simulink model "TorqueVect"  (R2022a)
settings: Solver=VariableStepAuto  StartTime=0.0  StopTime=300  RelTol=1e-3
PreLoadFcn:
  | run('Parameters\FSE_Parameters.m')
values from neighbouring files (symbols this model uses):
  Kd = 0;')    [open_carmaker_gui.m]
  Ki = 0    [open_carmaker_gui.m]
undefined symbols (not defined in the file or in its folder): BRegenEnabledButton, canChannel, CyalphaLookUp, efficiency, Fz_curve, Fz_scaling_long, gearR, izz, jw, kd, ki, Kp, kp, l_f, l_r, lambda, m, Mz_max, N, N_lat, N_long, P_max, pid_kd_lat, pid_kd_long, pid_ki_lat, pid_ki_long, pid_kp_lat, pid_kp_long, R_max, rw, steerR, T_i_max, TC_Decr_Gas, TC_Derivative, TC_Incr_Gas, TC_On, TC_Relay_Off, TC_Relay_On, tireCornerStiffness, Ts, TV_On, TV_Override, velocity_lookup, velocity_lookup_lat, y_ref, yrr_scaling
libraries: simulink x218, slpidlib x135, CarMaker4SL x73, TractionControlLibrary x13, canmsglib x9, canlib x8, TorqueVectoringLibrary x6, simulink_extras x4, PedalConversionLibrary x3, PowerControlLibrary x1
(part 7 of 26)

== system TorqueVect/CarMaker/IPG Vehicle/PowerTrain/PTControl Example/PTControl_ALL_CTRL_VC_MFE24/New TC/TC R3 ==
  modified slip ratio reference : Inport
  lim 1 : Inport  Port=2
  modified slip ratio measurement : Inport  Port=3
  P_TC : Inport  Port=4
  D_TC : Inport  Port=5
  enable_tc : Inport  Port=6
  PID Controller : slpidlib/PID Controller  Commented=on  Controller=PD  Form=Parallel  TimeDomain=Discrete-time  UseExternalTs=off  SampleTime=-1  IntegratorMethod=Forward Euler  FilterMethod=Forward Euler  ControllerParametersSource=external  P=125  I=1  UseKiTs=on  D=0  N=100  UseFilter=on  TunerSelectOption=Transfer Function Based (PID Tuner App)  InitialConditionSource=internal  InitialConditionForIntegrator=0  InitialConditionForFilter=0  DifferentiatorICPrevScaledInput=0  ExternalReset=none  TrackingMode=off  Kt=1  LimitOutput=on  SatLimitsSource=external  UpperSaturationLimit=inf  LowerSaturationLimit=-inf  LinearizeAsGain=on  AntiWindupMode=clamping  Kb=1  POutMin=[]  POutMax=[]  IOutMin=[]  IOutMax=[]  DOutMin=[]  DOutMax=[]  NOutMin=[]  NOutMax=[]  SumOutMin=[]  SumOutMax=[]  SaturationOutMin=[]  SaturationOutMax=[]  PParamMin=[]  PParamMax=[]  IParamMin=[]  IParamMax=[]  DParamMin=[]  DParamMax=[]  NParamMin=[]  NParamMax=[]  KbParamMin=[]  KbParamMax=[]  KtParamMin=[]  KtParamMax=[]  KbOutMin=[]  KbOutMax=[]  KtOutMin=[]  KtOutMax=[]  IntegratorOutMin=[]  IntegratorOutMax=[]  FilterOutMin=[]  FilterOutMax=[]  SumI1OutMin=[]  SumI1OutMax=[]  SumI2OutMin=[]  SumI2OutMax=[]  SumI3OutMin=[]  SumI3OutMax=[]  SumI4OutMin=[]  SumI4OutMax=[]  SumDOutMin=[]  SumDOutMax=[]  DifferentiatorOutMin=[]  DifferentiatorOutMax=[]  FilterDiffOutCoefMin=[]  FilterDiffOutCoefMax=[]  ReciprocalOutMin=[]  ReciprocalOutMax=[]  SumDenOutMin=[]  SumDenOutMax=[]  SumNumOutMin=[]  SumNumOutMax=[]  DivideOutMin=[]  DivideOutMax=[]  UdiffTsProdOutMin=[]  UdiffTsProdOutMax=[]  NTsProdOutMin=[]  NTsProdOutMax=[]  UintegralTsProdOutMin=[]  UintegralTsProdOutMax=[]  UngainTsProdOutMin=[]  UngainTsProdOutMax=[]  ClampingZeroOutDataTypeStr=Inherit: Inherit via back propagation  ClampingZeroOutMin=[]  ClampingZeroOutMax=[]  FilterDenConstantOutDataTypeStr=Inherit: Inherit via back propagation  FilterDenConstantOutMin=[]  FilterDenConstantOutMax=[]  PCopyOutDataTypeStr=Inherit: Inherit via back propagation  PCopyOutMin=[]  PCopyOutMax=[]  NCopyOutDataTypeStr=Inherit: Inherit via back propagation  NCopyOutMin=[]  NCopyOutMax=[]  IntegratorContinuousStateAttributes=''  IntegratorStateMustResolveToSignalObject=off  IntegratorRTWStateStorageClass=Auto  FilterContinuousStateAttributes=''  FilterStateMustResolveToSignalObject=off  FilterRTWStateStorageClass=Auto  ParallelPVariant=ExternalParameters  IdealPVariant=Disabled  IVariant=Disabled  DVariant=ExternalParameters  IntegratorVariant=Disabled  SatVariant=External  AWVariant=Disabled  PCopyVariant=Disabled  TRVariant=Disabled  FdbkBlocksVariant=Forward  IdealPFdbkVariant=Disabled  SatFdbkVariant=Disabled  DerivativeFilterVariant=ForwardEulerFilter  NVariant=ExternalParameters  NCopyVariant=Disabled  FilterICVariant=InternalICsFilter  IntegratorICVariant=Disabled  ExternalResetVariant=Disabled  TRSumVariant=Passthrough  SumFdbkVariant=Disabled  SumVariant=Sum_PD  TsampFilterVariant=InternalTs  TsampNgainVariant=Passthrough  TsampIntegralVariant=Disabled_SignalSpec  ExternalSaturationOutDataTypeStr=Inherit: Same as second input  aMode=0
  Sum1 : Sum  Inputs=|-+
  Sum2 : Sum  Commented=on  Inputs=|-+
  traction_controller : Subsystem
  Control Effort 1 : Outport
  wires:
  modified slip ratio reference/1 -> Sum1/1
  modified slip ratio measurement/1 -> Sum1/2
  lim 1/1 -> Sum2/2, traction_controller/1(max_torque)
  PID Controller/1 -> Sum2/1
  traction_controller/1(delta_torque) -> Control Effort 1/1
  enable_tc/1 -> traction_controller/3(enable_tc)
  Sum1/1 -> traction_controller/2(dslip)
  P_TC/1 -> traction_controller/4(Kp)
  D_TC/1 -> traction_controller/5(Kd)

== system TorqueVect/CarMaker/IPG Vehicle/PowerTrain/PTControl Example/PTControl_ALL_CTRL_VC_MFE24/New TC/TC R4 ==
  modified slip ratio reference : Inport
  lim 1 : Inport  Port=2
  modified slip ratio measurement : Inport  Port=3
  P_TC : Inport  Port=4
  D_TC : Inport  Port=5
  enable_tc : Inport  Port=6
  PID Controller : slpidlib/PID Controller  Commented=on  Controller=PD  Form=Parallel  TimeDomain=Discrete-time  UseExternalTs=off  SampleTime=-1  IntegratorMethod=Forward Euler  FilterMethod=Forward Euler  ControllerParametersSource=external  P=125  I=1  UseKiTs=on  D=0  N=100  UseFilter=on  TunerSelectOption=Transfer Function Based (PID Tuner App)  InitialConditionSource=internal  InitialConditionForIntegrator=0  InitialConditionForFilter=0  DifferentiatorICPrevScaledInput=0  ExternalReset=none  TrackingMode=off  Kt=1  LimitOutput=on  SatLimitsSource=external  UpperSaturationLimit=inf  LowerSaturationLimit=-inf  LinearizeAsGain=on  AntiWindupMode=clamping  Kb=1  POutMin=[]  POutMax=[]  IOutMin=[]  IOutMax=[]  DOutMin=[]  DOutMax=[]  NOutMin=[]  NOutMax=[]  SumOutMin=[]  SumOutMax=[]  SaturationOutMin=[]  SaturationOutMax=[]  PParamMin=[]  PParamMax=[]  IParamMin=[]  IParamMax=[]  DParamMin=[]  DParamMax=[]  NParamMin=[]  NParamMax=[]  KbParamMin=[]  KbParamMax=[]  KtParamMin=[]  KtParamMax=[]  KbOutMin=[]  KbOutMax=[]  KtOutMin=[]  KtOutMax=[]  IntegratorOutMin=[]  IntegratorOutMax=[]  FilterOutMin=[]  FilterOutMax=[]  SumI1OutMin=[]  SumI1OutMax=[]  SumI2OutMin=[]  SumI2OutMax=[]  SumI3OutMin=[]  SumI3OutMax=[]  SumI4OutMin=[]  SumI4OutMax=[]  SumDOutMin=[]  SumDOutMax=[]  DifferentiatorOutMin=[]  DifferentiatorOutMax=[]  FilterDiffOutCoefMin=[]  FilterDiffOutCoefMax=[]  ReciprocalOutMin=[]  ReciprocalOutMax=[]  SumDenOutMin=[]  SumDenOutMax=[]  SumNumOutMin=[]  SumNumOutMax=[]  DivideOutMin=[]  DivideOutMax=[]  UdiffTsProdOutMin=[]  UdiffTsProdOutMax=[]  NTsProdOutMin=[]  NTsProdOutMax=[]  UintegralTsProdOutMin=[]  UintegralTsProdOutMax=[]  UngainTsProdOutMin=[]  UngainTsProdOutMax=[]  ClampingZeroOutDataTypeStr=Inherit: Inherit via back propagation  ClampingZeroOutMin=[]  ClampingZeroOutMax=[]  FilterDenConstantOutDataTypeStr=Inherit: Inherit via back propagation  FilterDenConstantOutMin=[]  FilterDenConstantOutMax=[]  PCopyOutDataTypeStr=Inherit: Inherit via back propagation  PCopyOutMin=[]  PCopyOutMax=[]  NCopyOutDataTypeStr=Inherit: Inherit via back propagation  NCopyOutMin=[]  NCopyOutMax=[]  IntegratorContinuousStateAttributes=''  IntegratorStateMustResolveToSignalObject=off  IntegratorRTWStateStorageClass=Auto  FilterContinuousStateAttributes=''  FilterStateMustResolveToSignalObject=off  FilterRTWStateStorageClass=Auto  ParallelPVariant=ExternalParameters  IdealPVariant=Disabled  IVariant=Disabled  DVariant=ExternalParameters  IntegratorVariant=Disabled  SatVariant=External  AWVariant=Disabled  PCopyVariant=Disabled  TRVariant=Disabled  FdbkBlocksVariant=Forward  IdealPFdbkVariant=Disabled  SatFdbkVariant=Disabled  DerivativeFilterVariant=ForwardEulerFilter  NVariant=ExternalParameters  NCopyVariant=Disabled  FilterICVariant=InternalICsFilter  IntegratorICVariant=Disabled  ExternalResetVariant=Disabled  TRSumVariant=Passthrough  SumFdbkVariant=Disabled  SumVariant=Sum_PD  TsampFilterVariant=InternalTs  TsampNgainVariant=Passthrough  TsampIntegralVariant=Disabled_SignalSpec  ExternalSaturationOutDataTypeStr=Inherit: Same as second input  aMode=0
  Sum1 : Sum  Inputs=|-+
  Sum2 : Sum  Commented=on  Inputs=|-+
  traction_controller : Subsystem
  Control Effort 1 : Outport
  wires:
  modified slip ratio reference/1 -> Sum1/1
  modified slip ratio measurement/1 -> Sum1/2
  lim 1/1 -> Sum2/2, traction_controller/1(max_torque)
  PID Controller/1 -> Sum2/1
  traction_controller/1(delta_torque) -> Control Effort 1/1
  enable_tc/1 -> traction_controller/3(enable_tc)
  Sum1/1 -> traction_controller/2(dslip)
  P_TC/1 -> traction_controller/4(Kp)
  D_TC/1 -> traction_controller/5(Kd)

== system TorqueVect/CarMaker/IPG Vehicle/PowerTrain/PTControl Example/PTControl_ALL_CTRL_VC_MFE24/Subsystem/PedalConversion ==
  rThrottlePedal : Inport  OutMin=0  OutMax=1  PortDimensions=1
      settings: AttributesFormatString=[%<OutMin>, %<OutMax>]
  rLimitThrottleHigh : Inport  Port=2
  rLimitThrottleLow : Inport  Port=3
  BRegenEnable : Inport  Port=4
  vLong : Inport  Port=5
  1-D Lookup Table : Lookup_n-D  NumberOfTableDimensions=1  BreakpointsForDimension1=[0 0.3 0.35 1]  Table=[-1 0 0 1]  InternalRulePriority=Speed  RndMeth=Simplest
  AND : Logic  IconShape=distinctive  AllPortsSameDT=off  OutDataTypeStr=boolean
  Compare To Constant : simulink/Logic and Bit Operations/Compare To Constant  relop=>  const=5.0  OutDataTypeStr=boolean
  Rate Limiter Dynamic : simulink/Discontinuities/Rate Limiter Dynamic
  Saturation : Saturate  UpperLimit=1  LowerLimit=-1  OutMin=-1  OutMax=1
      settings: AttributesFormatString=[%<LowerLimit>, %<UpperLimit>]
  Saturation1 : Saturate  UpperLimit=1  LowerLimit=0  OutMin=-1  OutMax=1
      settings: AttributesFormatString=[%<LowerLimit>, %<UpperLimit>]
  Switch : Switch  Criteria=u2 > Threshold  SaturateOnIntegerOverflow=off  InputSameDT=off
  rThrottle : Outport  OutMin=-1  OutMax=1
      settings: AttributesFormatString=[%<OutMin>, %<OutMax>]
  wires:
  rLimitThrottleHigh/1 -> Rate Limiter Dynamic/1
  rLimitThrottleLow/1 -> Rate Limiter Dynamic/3
  Saturation/1 -> Switch/1
  Saturation1/1 -> Switch/3
  Switch/1 -> rThrottle/1
  rThrottlePedal/1 -> Rate Limiter Dynamic/2
  1-D Lookup Table/1 -> Saturation/1, Saturation1/1
  Rate Limiter Dynamic/1 -> 1-D Lookup Table/1
  AND/1 -> Switch/2
  BRegenEnable/1 -> AND/1
  vLong/1 -> Compare To Constant/1
  Compare To Constant/1 -> AND/2

== system TorqueVect/CarMaker/IPG Vehicle/PowerTrain/PTControl Example/PTControl_ALL_CTRL_VC_MFE24/Subsystem/PowerControl1 ==
  PMeasured : Inport  OutMin=-250000  OutMax=250000  Unit=W  PortDimensions=1
      settings: AttributesFormatString=[%<OutMin>, %<OutMax>] %<Unit>
  rSplitF : Inport  Port=2  OutMin=0  OutMax=1  PortDimensions=1
      settings: AttributesFormatString=[%<OutMin>, %<OutMax>]
  rThrottlePedal : Inport  Port=3  OutMin=0  OutMax=1  PortDimensions=1
      settings: AttributesFormatString=[%<OutMin>, %<OutMax>]
  PLimit : Inport  Port=4  OutMin=0  OutMax=80000  Unit=W  PortDimensions=1
      settings: AttributesFormatString=[%<OutMin>, %<OutMax>] %<Unit>
  FF_PC : Inport  Port=5
  P_PC : Inport  Port=6
  D_PC : Inport  Port=7
  I_PC : Inport  Port=8
  MMotorMax : Inport  Port=9
  rThrottle : Inport  Port=10
  FF_RC : Inport  Port=11
  PRegenLimit : Inport  Port=12
  BRegenEnable : Inport  Port=13
  P_RC : Inport  Port=14
  D_RC : Inport  Port=15
  I_RC : Inport  Port=16
  MRegenMotorMax : Inport  Port=17
  Add : Sum
  Constant : Constant  Value=0
  Constant1 : Constant  Value=0
  Gain : Gain  Gain=0.5
  Gain1 : Gain  Gain=0.5
  PC PID : Subsystem
  PID1 : Subsystem  Commented=on
  PowerError : Subsystem
  RC PID : Subsystem
  RegenError : Subsystem
  ResetPID_PC : Subsystem
  ResetPID_RC : Subsystem
  Subsystem : Subsystem
  TotalPower : Subsystem
  Unit Delay : UnitDelay  SampleTime=-1  HasFrameUpgradeWarning=on
  Unit Delay1 : UnitDelay  SampleTime=-1  HasFrameUpgradeWarning=on
  MChangeMotorFL : Outport  OutMin=-21  OutMax=21  Unit=N*m  PortDimensions=1
      settings: AttributesFormatString=[%<OutMin>, %<OutMax>] %<Unit>
  MChangeMotorFR : Outport  Port=2  OutMin=-21  OutMax=21  Unit=N*m  PortDimensions=1
      settings: AttributesFormatString=[%<OutMin>, %<OutMax>] %<Unit>
  MChangeMotorRL : Outport  Port=3  OutMin=-21  OutMax=21  Unit=N*m  PortDimensions=1
      settings: AttributesFormatString=[%<OutMin>, %<OutMax>] %<Unit>
  MChangeMotorRR : Outport  Port=4  OutMin=-21  OutMax=21  Unit=N*m  PortDimensions=1
      settings: AttributesFormatString=[%<OutMin>, %<OutMax>] %<Unit>
  PError : Outport  Port=5
  PRegenError : Outport  Port=6
  PPositiveTotal : Outport  Port=7
  PTotal : Outport  Port=8
  wires:
  Unit Delay/1 -> ResetPID_PC/2(PReductionTotal)
  Subsystem/1(TrqReductionR) -> Gain/1
  Subsystem/2(TrqReductionF) -> Gain1/1
  rSplitF/1 -> Subsystem/2(rSplitF)
  Gain/1 -> MChangeMotorRL/1, MChangeMotorRR/1
  Gain1/1 -> MChangeMotorFL/1, MChangeMotorFR/1
  PowerError/1(PError) -> PError/1, PC PID/1(PError)  "PError"
  FF_PC/1 -> PowerError/2(FF_PC)
  PLimit/1 -> PowerError/3(PLimit)
  P_PC/1 -> PC PID/2(P_PC)
  D_PC/1 -> PC PID/3(D_PC)
  I_PC/1 -> PC PID/4(I_PC)
  MMotorMax/1 -> PC PID/6(MMotorMax)
  MRegenMotorMax/1 -> RC PID/6(MRegenMotorMax)
  RegenError/1(PRegenError) -> PRegenError/1, RC PID/1(PRegenError)  "RegenError"
  BRegenEnable/1 -> ResetPID_RC/3(BRegenEnabled1), RegenError/5(BRegenEnable)
  rThrottle/1 -> RegenError/4(rThrottle)
  PRegenLimit/1 -> RegenError/3(PRegenLimit)
  FF_RC/1 -> RegenError/2(FF_RC)
  TotalPower/1(PPositiveTotal) -> PPositiveTotal/1, PowerError/1(PPositiveTotal)
  Add/1 -> Subsystem/1(TrqReductionTotal)
  PC PID/1(TrqReductionTotal) -> Unit Delay/1, Add/1
  RC PID/1(RegenTrqReductionTotal) -> Add/2, Unit Delay1/1
  Unit Delay1/1 -> ResetPID_RC/2(RegenTrqReductionTotal1)
  rThrottlePedal/1 -> [rThrottlePedal]
  [rThrottlePedal] -> ResetPID_PC/1(rThrottlePedal)
  [rThrottlePedal] -> ResetPID_RC/1(rThrottlePedal1)
  P_RC/1 -> RC PID/2(P_RC)
  D_RC/1 -> RC PID/3(D_RC)
  I_RC/1 -> RC PID/4(I_RC)
  PMeasured/1 -> TotalPower/1(PMeasured)
  TotalPower/2(PTotal) -> PTotal/1, ResetPID_RC/4(Current), RegenError/1(PTotal)
  Constant/1 -> RC PID/5(ResetPID_RC)
  Constant1/1 -> PC PID/5(ResetPID_PC)

== system TorqueVect/CarMaker/IPG Vehicle/PowerTrain/PTControl Example/PTControl_ALL_CTRL_VC_MFE24/Subsystem/PowerControl2 ==
  MMotorFL : Inport  OutMin=-42  OutMax=42  Unit=N*m  PortDimensions=1
      settings: AttributesFormatString=[%<OutMin>, %<OutMax>] %<Unit>
  MMotorFR : Inport  Port=2  OutMin=-42  OutMax=42  Unit=N*m  PortDimensions=1
      settings: AttributesFormatString=[%<OutMin>, %<OutMax>] %<Unit>
  MMotorRL : Inport  Port=3  OutMin=-42  OutMax=42  Unit=N*m  PortDimensions=1
      settings: AttributesFormatString=[%<OutMin>, %<OutMax>] %<Unit>
  MMotorRR : Inport  Port=4  OutMin=-42  OutMax=42  Unit=N*m  PortDimensions=1
      settings: AttributesFormatString=[%<OutMin>, %<OutMax>] %<Unit>
  nMotorFL : Inport  Port=5  OutMin=-3000  OutMax=3000  Unit=rad/s  PortDimensions=1
      settings: AttributesFormatString=[%<OutMin>, %<OutMax>] %<Unit>
  nMotorFR : Inport  Port=6  OutMin=-3000  OutMax=3000  Unit=rad/s  PortDimensions=1
      settings: AttributesFormatString=[%<OutMin>, %<OutMax>] %<Unit>
  nMotorRL : Inport  Port=7  OutMin=-3000  OutMax=3000  Unit=rad/s  PortDimensions=1
      settings: AttributesFormatString=[%<OutMin>, %<OutMax>] %<Unit>
  nMotorRR : Inport  Port=8  OutMin=-3000  OutMax=3000  Unit=rad/s  PortDimensions=1
      settings: AttributesFormatString=[%<OutMin>, %<OutMax>] %<Unit>
  PMeasured : Inport  Port=9  OutMin=-250000  OutMax=250000  Unit=W  PortDimensions=1
      settings: AttributesFormatString=[%<OutMin>, %<OutMax>] %<Unit>
  BMeasuredEnable : Inport  Port=10  OutMin=0  OutMax=1  PortDimensions=1
      settings: AttributesFormatString=[%<OutMin> / %<OutMax>]
  rSplitF : Inport  Port=11  OutMin=0  OutMax=1  PortDimensions=1
      settings: AttributesFormatString=[%<OutMin>, %<OutMax>]
  rThrottlePedal : Inport  Port=12  OutMin=0  OutMax=1  PortDimensions=1
      settings: AttributesFormatString=[%<OutMin>, %<OutMax>]
  PLimit : Inport  Port=13  OutMin=0  OutMax=80000  Unit=W  PortDimensions=1
      settings: AttributesFormatString=[%<OutMin>, %<OutMax>] %<Unit>
  FF_PC : Inport  Port=14
  P_PC : Inport  Port=15
  D_PC : Inport  Port=16
  I_PC : Inport  Port=17
  MMotorMax : Inport  Port=18
  rThrottle : Inport  Port=19
  FF_RC : Inport  Port=20
  PRegenLimit : Inport  Port=21
  BRegenEnable : Inport  Port=22
  P_RC : Inport  Port=23
  D_RC : Inport  Port=24
  I_RC : Inport  Port=25
  MRegenMotorMax : Inport  Port=26
  Add : Sum
  Gain : Gain  Gain=0.5
  Gain1 : Gain  Gain=0.5
  PC PID : Subsystem
  PID1 : Subsystem  Commented=on
  PowerError : Subsystem
  RC PID : Subsystem
  RegenError : Subsystem
  ResetPID_PC : Subsystem
  ResetPID_RC : Subsystem
  Subsystem : Subsystem
  TotalPower : Subsystem
  Unit Delay : UnitDelay  SampleTime=-1  HasFrameUpgradeWarning=on
  Unit Delay1 : UnitDelay  SampleTime=-1  HasFrameUpgradeWarning=on
  MChangeMotorFL : Outport  OutMin=-21  OutMax=21  Unit=N*m  PortDimensions=1
      settings: AttributesFormatString=[%<OutMin>, %<OutMax>] %<Unit>
  MChangeMotorFR : Outport  Port=2  OutMin=-21  OutMax=21  Unit=N*m  PortDimensions=1
      settings: AttributesFormatString=[%<OutMin>, %<OutMax>] %<Unit>
  MChangeMotorRL : Outport  Port=3  OutMin=-21  OutMax=21  Unit=N*m  PortDimensions=1
      settings: AttributesFormatString=[%<OutMin>, %<OutMax>] %<Unit>
  MChangeMotorRR : Outport  Port=4  OutMin=-21  OutMax=21  Unit=N*m  PortDimensions=1
      settings: AttributesFormatString=[%<OutMin>, %<OutMax>] %<Unit>
  PError : Outport  Port=5
  PRegenError : Outport  Port=6
  PPositiveTotal : Outport  Port=7
  PTotal : Outport  Port=8
  wires:
  Unit Delay/1 -> ResetPID_PC/2(PReductionTotal)
  Subsystem/1(TrqReductionR) -> Gain/1
  Subsystem/2(TrqReductionF) -> Gain1/1
  rSplitF/1 -> Subsystem/2(rSplitF)
  Gain/1 -> MChangeMotorRL/1, MChangeMotorRR/1
  Gain1/1 -> MChangeMotorFL/1, MChangeMotorFR/1
  PowerError/1(PError) -> PError/1, PC PID/1(PError)
  FF_PC/1 -> PowerError/2(FF_PC)
  PLimit/1 -> PowerError/3(PLimit)
  P_PC/1 -> PC PID/2(P_PC)
  D_PC/1 -> PC PID/3(D_PC)
  I_PC/1 -> PC PID/4(I_PC)
  MMotorMax/1 -> PC PID/6(MMotorMax)
  MRegenMotorMax/1 -> RC PID/6(MRegenMotorMax)
  RegenError/1(PRegenError) -> PRegenError/1, RC PID/1(PRegenError)
  BRegenEnable/1 -> RegenError/5(BRegenEnable), ResetPID_RC/3(BRegenEnabled)
  rThrottle/1 -> RegenError/4(rThrottle)
  PRegenLimit/1 -> RegenError/3(PRegenLimit)
  FF_RC/1 -> RegenError/2(FF_RC)
  TotalPower/1(PPositiveTotal) -> PPositiveTotal/1, PowerError/1(PPositiveTotal)
  Add/1 -> Subsystem/1(TrqReductionTotal)
  PC PID/1(TrqReductionTotal) -> Unit Delay/1, Add/1
  RC PID/1(RegenTrqReductionTotal) -> Unit Delay1/1, Add/2
  ResetPID_PC/1(ResetPID_PC) -> PC PID/5(ResetPID_PC)
  ResetPID_RC/1(ResetPID_RC) -> RC PID/5(ResetPID_RC)
  Unit Delay1/1 -> ResetPID_RC/2(RegenTrqReductionTotal)
  rThrottlePedal/1 -> [rThrottlePedal]
  [rThrottlePedal] -> ResetPID_PC/1(rThrottlePedal)
  [rThrottlePedal] -> ResetPID_RC/1(rThrottlePedal)
  P_RC/1 -> RC PID/2(P_RC)
  D_RC/1 -> RC PID/3(D_RC)
  I_RC/1 -> RC PID/4(I_RC)
  PMeasured/1 -> TotalPower/9(PMeasured)
  MMotorRL/1 -> TotalPower/5(MMotorRL)
  MMotorFL/1 -> TotalPower/1(MMotorFL)
  TotalPower/2(PTotal) -> PTotal/1, RegenError/1(PTotal), ResetPID_RC/4(PTotal)
  nMotorRL/1 -> TotalPower/6(nMotorRL)
  nMotorFR/1 -> TotalPower/4(nMotorFR)
  MMotorRR/1 -> TotalPower/7(MMotorRR)
  nMotorFL/1 -> TotalPower/2(nMotorFL)
  nMotorRR/1 -> TotalPower/8(nMotorRR)
  MMotorFR/1 -> TotalPower/3(MMotorFR)
  BMeasuredEnable/1 -> TotalPower/10(BMeasuredEnable)

== system TorqueVect/CarMaker/IPG Vehicle/PowerTrain/PTControl Example/PTControl_ALL_CTRL_VC_MFE24/Subsystem/Rate Limiter ==
  MMotorDemandedFL : Inport
  MMotorDemandedFR : Inport  Port=2
  MMotorDemandedRL : Inport  Port=3
  MMotorDemandedRR : Inport  Port=4
  rThrottle : Inport  Port=5
  rLimitHigh : Inport  Port=6
  rLimitLow : Inport  Port=7
  rLimitRegenHigh : Inport  Port=8
  rLimitRegenLow : Inport  Port=9
  Rate Limiter Dynamic{1..4} (4 alike) : simulink/Discontinuities/Rate Limiter Dynamic
  Switch : Switch  SaturateOnIntegerOverflow=off  InputSameDT=off
  Switch1 : Switch  SaturateOnIntegerOverflow=off  InputSameDT=off
  MMotorDemandFL : Outport
  MMotorDemandFR : Outport  Port=2
  MMotorDemandRL : Outport  Port=3
  MMotorDemandRR : Outport  Port=4
  wires:
  Switch1/1 -> Rate Limiter Dynamic1/3, Rate Limiter Dynamic2/3, Rate Limiter Dynamic3/3, Rate Limiter Dynamic4/3
  rThrottle/1 -> Switch1/2, Switch/2
  rLimitHigh/1 -> Switch/1
  rLimitRegenHigh/1 -> Switch/3
  Switch/1 -> Rate Limiter Dynamic2/1, Rate Limiter Dynamic4/1, Rate Limiter Dynamic3/1, Rate Limiter Dynamic1/1
  rLimitLow/1 -> Switch1/1
  rLimitRegenLow/1 -> Switch1/3
  MMotorDemandedRR/1 -> Rate Limiter Dynamic4/2
  MMotorDemandedRL/1 -> Rate Limiter Dynamic3/2
  MMotorDemandedFR/1 -> Rate Limiter Dynamic2/2
  MMotorDemandedFL/1 -> Rate Limiter Dynamic1/2
  Rate Limiter Dynamic2/1 -> MMotorDemandFR/1
  Rate Limiter Dynamic1/1 -> MMotorDemandFL/1
  Rate Limiter Dynamic3/1 -> MMotorDemandRL/1
  Rate Limiter Dynamic4/1 -> MMotorDemandRR/1

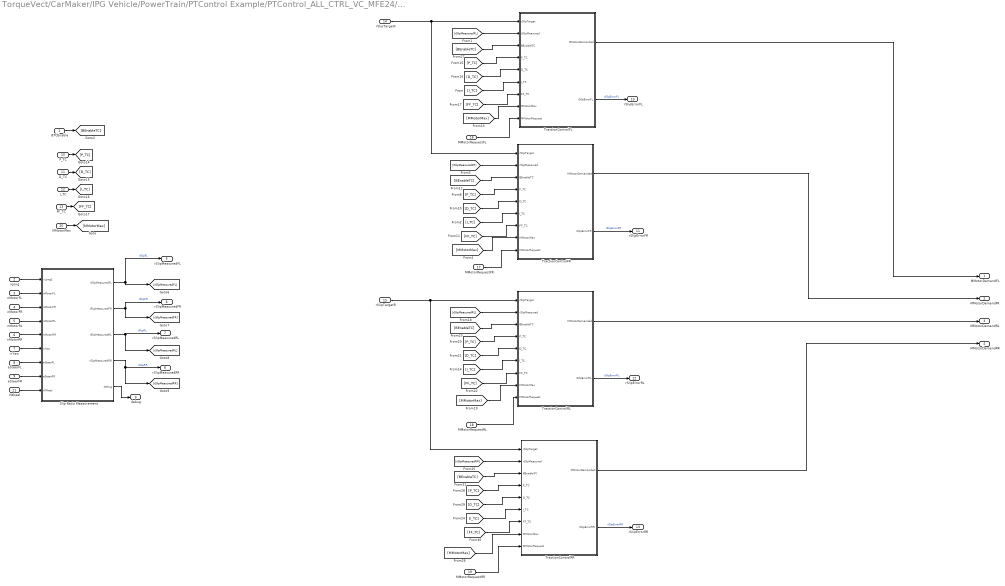
== system TorqueVect/CarMaker/IPG Vehicle/PowerTrain/PTControl Example/PTControl_ALL_CTRL_VC_MFE24/Subsystem/TC ==
  BTCEnable : Inport
  vLong : Inport  Port=2
  nMotorFL : Inport  Port=3  Unit=rad/s  PortDimensions=1
      settings: AttributesFormatString=%<Unit>
  nMotorFR : Inport  Port=4  Unit=rad/s  PortDimensions=1
      settings: AttributesFormatString=%<Unit>
  nMotorRL : Inport  Port=5  Unit=rad/s  PortDimensions=1
      settings: AttributesFormatString=%<Unit>
  nMotorRR : Inport  Port=6  Unit=rad/s  PortDimensions=1
      settings: AttributesFormatString=%<Unit>
  nYaw : Inport  Port=7
  aSteerFL : Inport  Port=8
  aSteerFR : Inport  Port=9
  P_TC : Inport  Port=10
  D_TC : Inport  Port=11
  I_TC : Inport  Port=12
  FF_TC : Inport  Port=13
  rSlipTargetF : Inport  Port=14
  rSlipTargetR : Inport  Port=15
  MMotorRequestFL : Inport  Port=16
  MMotorRequestFR : Inport  Port=17
  MMotorRequestRL : Inport  Port=18
  MMotorRequestRR : Inport  Port=19
  MMotorMax : Inport  Port=20
  rWheel : Inport  Port=21
  Slip Ratio Measurement : Subsystem
  TractionControlFL : Subsystem
  TractionControlFR : Subsystem
  TractionControlRL : Subsystem
  TractionControlRR : Subsystem
  MMotorDemandFL : Outport
  MMotorDemandFR : Outport  Port=2
  MMotorDemandRL : Outport  Port=3
  MMotorDemandRR : Outport  Port=4
  rSlipMeasuredFL : Outport  Port=5
  rSlipMeasuredFR : Outport  Port=6
  rSlipMeasuredRL : Outport  Port=7
  rSlipMeasuredRR : Outport  Port=8
  debug : Outport  Port=9
  rSlipErrorFL : Outport  Port=10
  rSlipErrorFR : Outport  Port=11
  rSlipErrorRL : Outport  Port=12
  rSlipErrorRR : Outport  Port=13
  wires:
  [BEnableTC] -> TractionControlFL/3(BEnableTC)
  rSlipTargetR/1 -> TractionControlRR/1(rSlipTarget), TractionControlRL/1(rSlipTarget)
  MMotorRequestFL/1 -> TractionControlFL/9(MMotorRequest)
  TractionControlFR/1(MMotorDemanded) -> MMotorDemandFR/1
  [I_TC] -> TractionControlFL/6(I_TC)
  [FF_TC] -> TractionControlFL/7(FF_TC)
  [D_TC] -> TractionControlFL/5(D_TC)
  FF_TC/1 -> [FF_TC]
  I_TC/1 -> [I_TC]
  TractionControlRL/1(MMotorDemanded) -> MMotorDemandRL/1
  TractionControlFL/1(MMotorDemanded) -> MMotorDemandFL/1
  P_TC/1 -> [P_TC]
  [P_TC] -> TractionControlFL/4(P_TC)
  TractionControlRR/1(MMotorDemanded) -> MMotorDemandRR/1
  MMotorRequestFR/1 -> TractionControlFR/9(MMotorRequest)
  MMotorRequestRR/1 -> TractionControlRR/9(MMotorRequest)
  D_TC/1 -> [D_TC]
  rSlipTargetF/1 -> TractionControlFR/1(rSlipTarget), TractionControlFL/1(rSlipTarget)
  MMotorRequestRL/1 -> TractionControlRL/9(MMotorRequest)
  Slip Ratio Measurement/3(rSlipMeasuredRL) -> [rSlipMeasuredRL], rSlipMeasuredRL/1  "rSlipRL"
  Slip Ratio Measurement/2(rSlipMeasuredFR) -> [rSlipMeasuredFR], rSlipMeasuredFR/1  "rSlipFR"
  aSteerFR/1 -> Slip Ratio Measurement/8(aSteerFR)
  nMotorFR/1 -> Slip Ratio Measurement/3(nMotorFR)
  nYaw/1 -> Slip Ratio Measurement/6(nYaw)
  nMotorRR/1 -> Slip Ratio Measurement/5(nMotorRR)
  aSteerFL/1 -> Slip Ratio Measurement/7(aSteerFL)
  nMotorRL/1 -> Slip Ratio Measurement/4(nMotorRL)
  nMotorFL/1 -> Slip Ratio Measurement/2(nMotorFL)
  Slip Ratio Measurement/4(rSlipMeasuredRR) -> [rSlipMeasuredRR], rSlipMeasuredRR/1  "rSlipRR"
  Slip Ratio Measurement/1(rSlipMeasuredFL) -> [rSlipMeasuredFL], rSlipMeasuredFL/1  "rSlipFL"
  vLong/1 -> Slip Ratio Measurement/1(vLong1)
  [rSlipMeasuredFL] -> TractionControlFL/2(rSlipMeasured)
  MMotorMax/1 -> [MMotorMax]
  [MMotorMax] -> TractionControlFL/8(MMotorMax)
  [FF_TC] -> TractionControlFR/7(FF_TC)
  [P_TC] -> TractionControlFR/4(P_TC)
  [BEnableTC] -> TractionControlFR/3(BEnableTC)
  [D_TC] -> TractionControlFR/5(D_TC)
  [MMotorMax] -> TractionControlFR/8(MMotorMax)
  [rSlipMeasuredFR] -> TractionControlFR/2(rSlipMeasured)
  [I_TC] -> TractionControlFR/6(I_TC)
  [FF_TC] -> TractionControlRL/7(FF_TC)
  [P_TC] -> TractionControlRL/4(P_TC)
  [BEnableTC] -> TractionControlRL/3(BEnableTC)
  [D_TC] -> TractionControlRL/5(D_TC)
  [MMotorMax] -> TractionControlRL/8(MMotorMax)
  [rSlipMeasuredRL] -> TractionControlRL/2(rSlipMeasured)
  [I_TC] -> TractionControlRL/6(I_TC)
  [FF_TC] -> TractionControlRR/7(FF_TC)
  [P_TC] -> TractionControlRR/4(P_TC)
  [BEnableTC] -> TractionControlRR/3(BEnableTC)
  [D_TC] -> TractionControlRR/5(D_TC)
  [MMotorMax] -> TractionControlRR/8(MMotorMax)
  [rSlipMeasuredRR] -> TractionControlRR/2(rSlipMeasured)
  [I_TC] -> TractionControlRR/6(I_TC)
  Slip Ratio Measurement/5(debug) -> debug/1
  TractionControlFL/2(rSlipErrorFL) -> rSlipErrorFL/1  "rSlipErrorFL"
  TractionControlFR/2(rSlipErrorFR) -> rSlipErrorFR/1  "rSlipErrorFR"
  TractionControlRL/2(rSlipErrorRL) -> rSlipErrorRL/1  "rSlipErrorRL"
  TractionControlRR/2(rSlipErrorRR) -> rSlipErrorRR/1  "rSlipErrorRR"
  BTCEnable/1 -> [BEnableTC]
  rWheel/1 -> Slip Ratio Measurement/9(rWheel)

== system TorqueVect/CarMaker/IPG Vehicle/PowerTrain/PTControl Example/PTControl_ALL_CTRL_VC_MFE24/Subsystem/Torque Modification1 ==
  MChangeMotorFL : Inport
  MChangeMotorFR : Inport  Port=2
  MChangeMotorRL : Inport  Port=3
  MChangeMotorRR : Inport  Port=4
  MDemandMotorFL : Inport  Port=5
  MDemandMotorFR : Inport  Port=6
  MDemandMotorRL : Inport  Port=7
  MDemandMotorRR : Inport  Port=8
  Add{,1..3} (4 alike) : Sum  Inputs=-+
  Saturation{,1..3} (4 alike) : Saturate  UpperLimit=21  LowerLimit=-21
  Torque Limit Check FL : Subsystem
  Torque Limit Check FR : Subsystem
  Torque Limit Check RL : Subsystem
  Torque Limit Check RR : Subsystem
  MTorqueModFL : Outport
  MTorqueModFR : Outport  Port=2
  MTorqueModRL : Outport  Port=3
  MTorqueModRR : Outport  Port=4
  wires:
  Add/1 -> Saturation/1
  Add2/1 -> Saturation2/1
  Add3/1 -> Saturation3/1
  MDemandMotorFL/1 -> Add2/2, Torque Limit Check FL/2(MDemandMotorFL)
  MDemandMotorFR/1 -> Add3/2, Torque Limit Check FR/2(MDemandMotorFR)
  MChangeMotorFR/1 -> Add3/1
  MChangeMotorFL/1 -> Add2/1
  MDemandMotorRR/1 -> Add1/2, Torque Limit Check RR/2(MDemandMotorRR)
  MChangeMotorRR/1 -> Add1/1
  MChangeMotorRL/1 -> Add/1
  MDemandMotorRL/1 -> Add/2, Torque Limit Check RL/2(MDemandMotorRL)
  Add1/1 -> Saturation1/1
  Saturation/1 -> Torque Limit Check RL/1(MTorqueNewRL)
  Torque Limit Check RL/1(MTorqueModRL) -> MTorqueModRL/1
  Torque Limit Check RR/1(MTorqueModRR) -> MTorqueModRR/1
  Saturation1/1 -> Torque Limit Check RR/1(MTorqueNewRR)
  Torque Limit Check FL/1(MTorqueModFL) -> MTorqueModFL/1
  Saturation2/1 -> Torque Limit Check FL/1(MTorqueNewFL)
  Torque Limit Check FR/1(MTorqueModFR) -> MTorqueModFR/1
  Saturation3/1 -> Torque Limit Check FR/1(MTorqueNewFR)

== system TorqueVect/CarMaker/IPG Vehicle/PowerTrain/PTControl Example/PTControl_ALL_CTRL_VC_MFE24/Subsystem/Torque Modification2 ==
  MChangeMotorFL : Inport
  MChangeMotorFR : Inport  Port=2
  MChangeMotorRL : Inport  Port=3
  MChangeMotorRR : Inport  Port=4
  MDemandMotorFL : Inport  Port=5
  MDemandMotorFR : Inport  Port=6
  MDemandMotorRL : Inport  Port=7
  MDemandMotorRR : Inport  Port=8
  Add{,1..3} (4 alike) : Sum  Inputs=-+
  Saturation{,1..3} (4 alike) : Saturate  UpperLimit=21  LowerLimit=-21
  Torque Limit Check FL : Subsystem
  Torque Limit Check FR : Subsystem
  Torque Limit Check RL : Subsystem
  Torque Limit Check RR : Subsystem
  MTorqueModFL : Outport
  MTorqueModFR : Outport  Port=2
  MTorqueModRL : Outport  Port=3
  MTorqueModRR : Outport  Port=4
  wires:
  Add/1 -> Saturation/1
  Add2/1 -> Saturation2/1
  Add3/1 -> Saturation3/1
  MDemandMotorFL/1 -> Add2/2, Torque Limit Check FL/2(MDemandMotorFL)
  MDemandMotorFR/1 -> Add3/2, Torque Limit Check FR/2(MDemandMotorFR)
  MChangeMotorFR/1 -> Add3/1
  MChangeMotorFL/1 -> Add2/1
  MDemandMotorRR/1 -> Add1/2, Torque Limit Check RR/2(MDemandMotorRR)
  MChangeMotorRR/1 -> Add1/1
  MChangeMotorRL/1 -> Add/1
  MDemandMotorRL/1 -> Add/2, Torque Limit Check RL/2(MDemandMotorRL)
  Add1/1 -> Saturation1/1
  Saturation/1 -> Torque Limit Check RL/1(MTorqueNewRL)
  Torque Limit Check RL/1(MTorqueModRL) -> MTorqueModRL/1
  Torque Limit Check RR/1(MTorqueModRR) -> MTorqueModRR/1
  Saturation1/1 -> Torque Limit Check RR/1(MTorqueNewRR)
  Torque Limit Check FL/1(MTorqueModFL) -> MTorqueModFL/1
  Saturation2/1 -> Torque Limit Check FL/1(MTorqueNewFL)
  Torque Limit Check FR/1(MTorqueModFR) -> MTorqueModFR/1
  Saturation3/1 -> Torque Limit Check FR/1(MTorqueNewFR)

== system TorqueVect/CarMaker/IPG Vehicle/PowerTrain/PTControl Example/PTControl_ALL_CTRL_VC_MFE24/Subsystem/Torque Vectoring ==
  BTVEnable : Inport
  aSlip : Inport  Port=2
  vLong : Inport  Port=3
  MMotorMax : Inport  Port=4
  NTorqueMaxDeltaF : Inport  Port=5
  NTorqueMaxDeltaR : Inport  Port=6
  P_YR : Inport  Port=7
  D_YR : Inport  Port=8
  I_YR : Inport  Port=9
  aSteer : Inport  Port=10
  MMotorDemandFL : Inport  Port=11
  MMotorDemandFR : Inport  Port=12
  MMotorDemandRL : Inport  Port=13
  MMotorDemandRR : Inport  Port=14
  Add : Sum
  Add1 : Sum
  Constant : Constant  Value=0.314159
  Constant1 : Constant  Value=3
  FPID : Subsystem
  RPID : Subsystem
  TV Enable Checker : Subsystem
  MMotorRequestFL : Outport
  MMotorRequestFR : Outport  Port=2
  MMotorRequestRL : Outport  Port=3
  MMotorRequestRR : Outport  Port=4
  wires:
  I_YR/1 -> [I_YR]
  D_YR/1 -> [D_YR]
  P_YR/1 -> [P_YR]
  MMotorMax/1 -> [MMotorMax]
  MMotorDemandRR/1 -> Add1/2
  MMotorDemandFR/1 -> Add/2
  MMotorDemandRL/1 -> Add1/1
  MMotorDemandFL/1 -> Add/1
  BTVEnable/1 -> TV Enable Checker/5(BTorqueVectoringEnable)
  aSlip/1 -> RPID/5(aSlip), FPID/5(aSlip)
  Add/1 -> FPID/4(NTorqueAxle)
  [MMotorMax] -> FPID/3(NTorqueMax)
  NTorqueMaxDeltaF/1 -> FPID/2(NTorqueMaxDelta)
  [P_YR] -> FPID/6(P_YR)
  [D_YR] -> FPID/7(D_YR)
  [I_YR] -> FPID/8(I_YR)
  FPID/2(NTorqueRightOut) -> MMotorRequestFR/1
  FPID/1(NTorqueLeftOut) -> MMotorRequestFL/1
  RPID/1(NTorqueLeftOut) -> MMotorRequestRL/1
  RPID/2(NTorqueRightOut) -> MMotorRequestRR/1
  NTorqueMaxDeltaR/1 -> RPID/2(NTorqueMaxDelta)
  [MMotorMax] -> RPID/3(NTorqueMax)
  [P_YR] -> RPID/6(P_YR)
  [D_YR] -> RPID/7(D_YR)
  [I_YR] -> RPID/8(I_YR)
  Add1/1 -> RPID/4(NTorqueAxle)
  aSteer/1 -> TV Enable Checker/2(aSteerWheel)
  Constant/1 -> TV Enable Checker/4(aSteerWheelMin)
  Constant1/1 -> TV Enable Checker/3(vLongMin)
  vLong/1 -> TV Enable Checker/1(vLong)
  TV Enable Checker/1(BEnable) -> RPID/1(BEnable), FPID/1(BEnable)  "Enable"

== system TorqueVect/CarMaker/IPG Vehicle/PowerTrain/PTControl Example/PTControl_ALL_CTRL_VC_MFE24/Subsystem/TorqueSplit ==
  rSplitF : Inport
  rThrottle : Inport  Port=2
  MMotorMax : Inport  Port=3
  MRegenMotorMax : Inport  Port=4
  Add : Sum  Inputs=-+
  Gain : Gain  Gain=4
  MATLAB Function : MATLAB Function  TreatAsAtomicUnit=on
  Product : Product
  Product1 : Product
  Switch : Switch  Criteria=u2 > Threshold  SaturateOnIntegerOverflow=off  InputSameDT=off
  MMotorDemandFL : Outport
  MMotorDemandFR : Outport  Port=2
  MMotorDemandRL : Outport  Port=3
  MMotorDemandRR : Outport  Port=4
  wires:
  MATLAB Function/4(rr_out) -> MMotorDemandRR/1
  MATLAB Function/3(rl_out) -> MMotorDemandRL/1
  Product1/1 -> MATLAB Function/1(f_in), Add/1
  rSplitF/1 -> Product1/1  "rSplitF"
  MATLAB Function/2(fr_out) -> MMotorDemandFR/1
  MATLAB Function/1(fl_out) -> MMotorDemandFL/1
  Product/1 -> Add/2, Product1/2
  Add/1 -> MATLAB Function/2(r_in)
  rThrottle/1 -> Switch/2, Product/2
  MMotorMax/1 -> Switch/1
  Gain/1 -> Product/1
  Switch/1 -> MATLAB Function/3(maxTrq), Gain/1
  MRegenMotorMax/1 -> Switch/3

== system TorqueVect/CarMaker/IPG Vehicle/PowerTrain/PTControl Example/PTControl_ALL_CTRL_VC_REGEN/New TC/Reference Generator1 ==
  note: Modified slip ratio targets
  note: Vehicle velocity
  note: For throttle sign and Product:
      | If positive, normal reference
      | If negative (regen), similar reference but negative (negative target slip*times speed), this might need to change to account for regen limits
      | If 0, target zero
  x2 : Inport
  Front SR Target : Inport  Port=2
  Rear SR Target : Inport  Port=3
  Constant : Constant
  Product1 : Product
  Product2 : Product
  Switch : Switch  Criteria=u2 > Threshold  Threshold=1  SaturateOnIntegerOverflow=off  InputSameDT=off
  R1 : Outport
  L1 : Outport  Port=2
  R2 : Outport  Port=3
  L2 : Outport  Port=4
  wires:
  Front SR Target/1 -> Product1/1
  Product1/1 -> L1/1, R1/1
  Product2/1 -> L2/1, R2/1
  Rear SR Target/1 -> Product2/2
  Switch/1 -> Product2/1, Product1/2
  x2/1 -> Switch/1, Switch/2
  Constant/1 -> Switch/3

== system TorqueVect/CarMaker/IPG Vehicle/PowerTrain/PTControl Example/PTControl_ALL_CTRL_VC_REGEN/New TC/TC R1 ==
  modified slip ratio reference : Inport
  lim 1 : Inport  Port=2
  modified slip ratio measurement : Inport  Port=3
  P_TC : Inport  Port=4
  D_TC : Inport  Port=5
  enable_tc : Inport  Port=6
  PID Controller : slpidlib/PID Controller  Commented=on  Controller=PD  Form=Parallel  TimeDomain=Discrete-time  UseExternalTs=off  SampleTime=-1  IntegratorMethod=Forward Euler  FilterMethod=Forward Euler  ControllerParametersSource=external  P=125  I=1  UseKiTs=on  D=0  N=100  UseFilter=on  TunerSelectOption=Transfer Function Based (PID Tuner App)  InitialConditionSource=internal  InitialConditionForIntegrator=0  InitialConditionForFilter=0  DifferentiatorICPrevScaledInput=0  ExternalReset=none  TrackingMode=off  Kt=1  LimitOutput=on  SatLimitsSource=external  UpperSaturationLimit=inf  LowerSaturationLimit=-inf  LinearizeAsGain=on  AntiWindupMode=clamping  Kb=1  POutMin=[]  POutMax=[]  IOutMin=[]  IOutMax=[]  DOutMin=[]  DOutMax=[]  NOutMin=[]  NOutMax=[]  SumOutMin=[]  SumOutMax=[]  SaturationOutMin=[]  SaturationOutMax=[]  PParamMin=[]  PParamMax=[]  IParamMin=[]  IParamMax=[]  DParamMin=[]  DParamMax=[]  NParamMin=[]  NParamMax=[]  KbParamMin=[]  KbParamMax=[]  KtParamMin=[]  KtParamMax=[]  KbOutMin=[]  KbOutMax=[]  KtOutMin=[]  KtOutMax=[]  IntegratorOutMin=[]  IntegratorOutMax=[]  FilterOutMin=[]  FilterOutMax=[]  SumI1OutMin=[]  SumI1OutMax=[]  SumI2OutMin=[]  SumI2OutMax=[]  SumI3OutMin=[]  SumI3OutMax=[]  SumI4OutMin=[]  SumI4OutMax=[]  SumDOutMin=[]  SumDOutMax=[]  DifferentiatorOutMin=[]  DifferentiatorOutMax=[]  FilterDiffOutCoefMin=[]  FilterDiffOutCoefMax=[]  ReciprocalOutMin=[]  ReciprocalOutMax=[]  SumDenOutMin=[]  SumDenOutMax=[]  SumNumOutMin=[]  SumNumOutMax=[]  DivideOutMin=[]  DivideOutMax=[]  UdiffTsProdOutMin=[]  UdiffTsProdOutMax=[]  NTsProdOutMin=[]  NTsProdOutMax=[]  UintegralTsProdOutMin=[]  UintegralTsProdOutMax=[]  UngainTsProdOutMin=[]  UngainTsProdOutMax=[]  ClampingZeroOutDataTypeStr=Inherit: Inherit via back propagation  ClampingZeroOutMin=[]  ClampingZeroOutMax=[]  FilterDenConstantOutDataTypeStr=Inherit: Inherit via back propagation  FilterDenConstantOutMin=[]  FilterDenConstantOutMax=[]  PCopyOutDataTypeStr=Inherit: Inherit via back propagation  PCopyOutMin=[]  PCopyOutMax=[]  NCopyOutDataTypeStr=Inherit: Inherit via back propagation  NCopyOutMin=[]  NCopyOutMax=[]  IntegratorContinuousStateAttributes=''  IntegratorStateMustResolveToSignalObject=off  IntegratorRTWStateStorageClass=Auto  FilterContinuousStateAttributes=''  FilterStateMustResolveToSignalObject=off  FilterRTWStateStorageClass=Auto  ParallelPVariant=ExternalParameters  IdealPVariant=Disabled  IVariant=Disabled  DVariant=ExternalParameters  IntegratorVariant=Disabled  SatVariant=External  AWVariant=Disabled  PCopyVariant=Disabled  TRVariant=Disabled  FdbkBlocksVariant=Forward  IdealPFdbkVariant=Disabled  SatFdbkVariant=Disabled  DerivativeFilterVariant=ForwardEulerFilter  NVariant=ExternalParameters  NCopyVariant=Disabled  FilterICVariant=InternalICsFilter  IntegratorICVariant=Disabled  ExternalResetVariant=Disabled  TRSumVariant=Passthrough  SumFdbkVariant=Disabled  SumVariant=Sum_PD  TsampFilterVariant=InternalTs  TsampNgainVariant=Passthrough  TsampIntegralVariant=Disabled_SignalSpec  ExternalSaturationOutDataTypeStr=Inherit: Same as second input  aMode=0
  Sum1 : Sum  Inputs=|-+
  Sum2 : Sum  Commented=on  Inputs=|-+
  traction_controller : Subsystem
  Control Effort 1 : Outport
  wires:
  modified slip ratio reference/1 -> Sum1/1
  modified slip ratio measurement/1 -> Sum1/2
  lim 1/1 -> Sum2/2, traction_controller/1(max_torque)
  PID Controller/1 -> Sum2/1
  traction_controller/1(delta_torque) -> Control Effort 1/1
  enable_tc/1 -> traction_controller/3(enable_tc)
  Sum1/1 -> traction_controller/2(dslip)
  P_TC/1 -> traction_controller/4(Kp)
  D_TC/1 -> traction_controller/5(Kd)

== system TorqueVect/CarMaker/IPG Vehicle/PowerTrain/PTControl Example/PTControl_ALL_CTRL_VC_REGEN/New TC/TC R2 ==
  modified slip ratio reference : Inport
  lim 1 : Inport  Port=2
  modified slip ratio measurement : Inport  Port=3
  P_TC : Inport  Port=4
  D_TC : Inport  Port=5
  enable_tc : Inport  Port=6
  PID Controller : slpidlib/PID Controller  Commented=on  Controller=PD  Form=Parallel  TimeDomain=Discrete-time  UseExternalTs=off  SampleTime=-1  IntegratorMethod=Forward Euler  FilterMethod=Forward Euler  ControllerParametersSource=external  P=125  I=1  UseKiTs=on  D=0  N=100  UseFilter=on  TunerSelectOption=Transfer Function Based (PID Tuner App)  InitialConditionSource=internal  InitialConditionForIntegrator=0  InitialConditionForFilter=0  DifferentiatorICPrevScaledInput=0  ExternalReset=none  TrackingMode=off  Kt=1  LimitOutput=on  SatLimitsSource=external  UpperSaturationLimit=inf  LowerSaturationLimit=-inf  LinearizeAsGain=on  AntiWindupMode=clamping  Kb=1  POutMin=[]  POutMax=[]  IOutMin=[]  IOutMax=[]  DOutMin=[]  DOutMax=[]  NOutMin=[]  NOutMax=[]  SumOutMin=[]  SumOutMax=[]  SaturationOutMin=[]  SaturationOutMax=[]  PParamMin=[]  PParamMax=[]  IParamMin=[]  IParamMax=[]  DParamMin=[]  DParamMax=[]  NParamMin=[]  NParamMax=[]  KbParamMin=[]  KbParamMax=[]  KtParamMin=[]  KtParamMax=[]  KbOutMin=[]  KbOutMax=[]  KtOutMin=[]  KtOutMax=[]  IntegratorOutMin=[]  IntegratorOutMax=[]  FilterOutMin=[]  FilterOutMax=[]  SumI1OutMin=[]  SumI1OutMax=[]  SumI2OutMin=[]  SumI2OutMax=[]  SumI3OutMin=[]  SumI3OutMax=[]  SumI4OutMin=[]  SumI4OutMax=[]  SumDOutMin=[]  SumDOutMax=[]  DifferentiatorOutMin=[]  DifferentiatorOutMax=[]  FilterDiffOutCoefMin=[]  FilterDiffOutCoefMax=[]  ReciprocalOutMin=[]  ReciprocalOutMax=[]  SumDenOutMin=[]  SumDenOutMax=[]  SumNumOutMin=[]  SumNumOutMax=[]  DivideOutMin=[]  DivideOutMax=[]  UdiffTsProdOutMin=[]  UdiffTsProdOutMax=[]  NTsProdOutMin=[]  NTsProdOutMax=[]  UintegralTsProdOutMin=[]  UintegralTsProdOutMax=[]  UngainTsProdOutMin=[]  UngainTsProdOutMax=[]  ClampingZeroOutDataTypeStr=Inherit: Inherit via back propagation  ClampingZeroOutMin=[]  ClampingZeroOutMax=[]  FilterDenConstantOutDataTypeStr=Inherit: Inherit via back propagation  FilterDenConstantOutMin=[]  FilterDenConstantOutMax=[]  PCopyOutDataTypeStr=Inherit: Inherit via back propagation  PCopyOutMin=[]  PCopyOutMax=[]  NCopyOutDataTypeStr=Inherit: Inherit via back propagation  NCopyOutMin=[]  NCopyOutMax=[]  IntegratorContinuousStateAttributes=''  IntegratorStateMustResolveToSignalObject=off  IntegratorRTWStateStorageClass=Auto  FilterContinuousStateAttributes=''  FilterStateMustResolveToSignalObject=off  FilterRTWStateStorageClass=Auto  ParallelPVariant=ExternalParameters  IdealPVariant=Disabled  IVariant=Disabled  DVariant=ExternalParameters  IntegratorVariant=Disabled  SatVariant=External  AWVariant=Disabled  PCopyVariant=Disabled  TRVariant=Disabled  FdbkBlocksVariant=Forward  IdealPFdbkVariant=Disabled  SatFdbkVariant=Disabled  DerivativeFilterVariant=ForwardEulerFilter  NVariant=ExternalParameters  NCopyVariant=Disabled  FilterICVariant=InternalICsFilter  IntegratorICVariant=Disabled  ExternalResetVariant=Disabled  TRSumVariant=Passthrough  SumFdbkVariant=Disabled  SumVariant=Sum_PD  TsampFilterVariant=InternalTs  TsampNgainVariant=Passthrough  TsampIntegralVariant=Disabled_SignalSpec  ExternalSaturationOutDataTypeStr=Inherit: Same as second input  aMode=0
  Sum1 : Sum  Inputs=|-+
  Sum2 : Sum  Commented=on  Inputs=|-+
  traction_controller : Subsystem
  Control Effort 1 : Outport
  wires:
  modified slip ratio reference/1 -> Sum1/1
  modified slip ratio measurement/1 -> Sum1/2
  lim 1/1 -> Sum2/2, traction_controller/1(max_torque)
  PID Controller/1 -> Sum2/1
  traction_controller/1(delta_torque) -> Control Effort 1/1
  enable_tc/1 -> traction_controller/3(enable_tc)
  Sum1/1 -> traction_controller/2(dslip)
  P_TC/1 -> traction_controller/4(Kp)
  D_TC/1 -> traction_controller/5(Kd)

== system TorqueVect/CarMaker/IPG Vehicle/PowerTrain/PTControl Example/PTControl_ALL_CTRL_VC_REGEN/New TC/TC R3 ==
  modified slip ratio reference : Inport
  lim 1 : Inport  Port=2
  modified slip ratio measurement : Inport  Port=3
  P_TC : Inport  Port=4
  D_TC : Inport  Port=5
  enable_tc : Inport  Port=6
  PID Controller : slpidlib/PID Controller  Commented=on  Controller=PD  Form=Parallel  TimeDomain=Discrete-time  UseExternalTs=off  SampleTime=-1  IntegratorMethod=Forward Euler  FilterMethod=Forward Euler  ControllerParametersSource=external  P=125  I=1  UseKiTs=on  D=0  N=100  UseFilter=on  TunerSelectOption=Transfer Function Based (PID Tuner App)  InitialConditionSource=internal  InitialConditionForIntegrator=0  InitialConditionForFilter=0  DifferentiatorICPrevScaledInput=0  ExternalReset=none  TrackingMode=off  Kt=1  LimitOutput=on  SatLimitsSource=external  UpperSaturationLimit=inf  LowerSaturationLimit=-inf  LinearizeAsGain=on  AntiWindupMode=clamping  Kb=1  POutMin=[]  POutMax=[]  IOutMin=[]  IOutMax=[]  DOutMin=[]  DOutMax=[]  NOutMin=[]  NOutMax=[]  SumOutMin=[]  SumOutMax=[]  SaturationOutMin=[]  SaturationOutMax=[]  PParamMin=[]  PParamMax=[]  IParamMin=[]  IParamMax=[]  DParamMin=[]  DParamMax=[]  NParamMin=[]  NParamMax=[]  KbParamMin=[]  KbParamMax=[]  KtParamMin=[]  KtParamMax=[]  KbOutMin=[]  KbOutMax=[]  KtOutMin=[]  KtOutMax=[]  IntegratorOutMin=[]  IntegratorOutMax=[]  FilterOutMin=[]  FilterOutMax=[]  SumI1OutMin=[]  SumI1OutMax=[]  SumI2OutMin=[]  SumI2OutMax=[]  SumI3OutMin=[]  SumI3OutMax=[]  SumI4OutMin=[]  SumI4OutMax=[]  SumDOutMin=[]  SumDOutMax=[]  DifferentiatorOutMin=[]  DifferentiatorOutMax=[]  FilterDiffOutCoefMin=[]  FilterDiffOutCoefMax=[]  ReciprocalOutMin=[]  ReciprocalOutMax=[]  SumDenOutMin=[]  SumDenOutMax=[]  SumNumOutMin=[]  SumNumOutMax=[]  DivideOutMin=[]  DivideOutMax=[]  UdiffTsProdOutMin=[]  UdiffTsProdOutMax=[]  NTsProdOutMin=[]  NTsProdOutMax=[]  UintegralTsProdOutMin=[]  UintegralTsProdOutMax=[]  UngainTsProdOutMin=[]  UngainTsProdOutMax=[]  ClampingZeroOutDataTypeStr=Inherit: Inherit via back propagation  ClampingZeroOutMin=[]  ClampingZeroOutMax=[]  FilterDenConstantOutDataTypeStr=Inherit: Inherit via back propagation  FilterDenConstantOutMin=[]  FilterDenConstantOutMax=[]  PCopyOutDataTypeStr=Inherit: Inherit via back propagation  PCopyOutMin=[]  PCopyOutMax=[]  NCopyOutDataTypeStr=Inherit: Inherit via back propagation  NCopyOutMin=[]  NCopyOutMax=[]  IntegratorContinuousStateAttributes=''  IntegratorStateMustResolveToSignalObject=off  IntegratorRTWStateStorageClass=Auto  FilterContinuousStateAttributes=''  FilterStateMustResolveToSignalObject=off  FilterRTWStateStorageClass=Auto  ParallelPVariant=ExternalParameters  IdealPVariant=Disabled  IVariant=Disabled  DVariant=ExternalParameters  IntegratorVariant=Disabled  SatVariant=External  AWVariant=Disabled  PCopyVariant=Disabled  TRVariant=Disabled  FdbkBlocksVariant=Forward  IdealPFdbkVariant=Disabled  SatFdbkVariant=Disabled  DerivativeFilterVariant=ForwardEulerFilter  NVariant=ExternalParameters  NCopyVariant=Disabled  FilterICVariant=InternalICsFilter  IntegratorICVariant=Disabled  ExternalResetVariant=Disabled  TRSumVariant=Passthrough  SumFdbkVariant=Disabled  SumVariant=Sum_PD  TsampFilterVariant=InternalTs  TsampNgainVariant=Passthrough  TsampIntegralVariant=Disabled_SignalSpec  ExternalSaturationOutDataTypeStr=Inherit: Same as second input  aMode=0
  Sum1 : Sum  Inputs=|-+
  Sum2 : Sum  Commented=on  Inputs=|-+
  traction_controller : Subsystem
  Control Effort 1 : Outport
  wires:
  modified slip ratio reference/1 -> Sum1/1
  modified slip ratio measurement/1 -> Sum1/2
  lim 1/1 -> Sum2/2, traction_controller/1(max_torque)
  PID Controller/1 -> Sum2/1
  traction_controller/1(delta_torque) -> Control Effort 1/1
  enable_tc/1 -> traction_controller/3(enable_tc)
  Sum1/1 -> traction_controller/2(dslip)
  P_TC/1 -> traction_controller/4(Kp)
  D_TC/1 -> traction_controller/5(Kd)

== system TorqueVect/CarMaker/IPG Vehicle/PowerTrain/PTControl Example/PTControl_ALL_CTRL_VC_REGEN/New TC/TC R4 ==
  modified slip ratio reference : Inport
  lim 1 : Inport  Port=2
  modified slip ratio measurement : Inport  Port=3
  P_TC : Inport  Port=4
  D_TC : Inport  Port=5
  enable_tc : Inport  Port=6
  PID Controller : slpidlib/PID Controller  Commented=on  Controller=PD  Form=Parallel  TimeDomain=Discrete-time  UseExternalTs=off  SampleTime=-1  IntegratorMethod=Forward Euler  FilterMethod=Forward Euler  ControllerParametersSource=external  P=125  I=1  UseKiTs=on  D=0  N=100  UseFilter=on  TunerSelectOption=Transfer Function Based (PID Tuner App)  InitialConditionSource=internal  InitialConditionForIntegrator=0  InitialConditionForFilter=0  DifferentiatorICPrevScaledInput=0  ExternalReset=none  TrackingMode=off  Kt=1  LimitOutput=on  SatLimitsSource=external  UpperSaturationLimit=inf  LowerSaturationLimit=-inf  LinearizeAsGain=on  AntiWindupMode=clamping  Kb=1  POutMin=[]  POutMax=[]  IOutMin=[]  IOutMax=[]  DOutMin=[]  DOutMax=[]  NOutMin=[]  NOutMax=[]  SumOutMin=[]  SumOutMax=[]  SaturationOutMin=[]  SaturationOutMax=[]  PParamMin=[]  PParamMax=[]  IParamMin=[]  IParamMax=[]  DParamMin=[]  DParamMax=[]  NParamMin=[]  NParamMax=[]  KbParamMin=[]  KbParamMax=[]  KtParamMin=[]  KtParamMax=[]  KbOutMin=[]  KbOutMax=[]  KtOutMin=[]  KtOutMax=[]  IntegratorOutMin=[]  IntegratorOutMax=[]  FilterOutMin=[]  FilterOutMax=[]  SumI1OutMin=[]  SumI1OutMax=[]  SumI2OutMin=[]  SumI2OutMax=[]  SumI3OutMin=[]  SumI3OutMax=[]  SumI4OutMin=[]  SumI4OutMax=[]  SumDOutMin=[]  SumDOutMax=[]  DifferentiatorOutMin=[]  DifferentiatorOutMax=[]  FilterDiffOutCoefMin=[]  FilterDiffOutCoefMax=[]  ReciprocalOutMin=[]  ReciprocalOutMax=[]  SumDenOutMin=[]  SumDenOutMax=[]  SumNumOutMin=[]  SumNumOutMax=[]  DivideOutMin=[]  DivideOutMax=[]  UdiffTsProdOutMin=[]  UdiffTsProdOutMax=[]  NTsProdOutMin=[]  NTsProdOutMax=[]  UintegralTsProdOutMin=[]  UintegralTsProdOutMax=[]  UngainTsProdOutMin=[]  UngainTsProdOutMax=[]  ClampingZeroOutDataTypeStr=Inherit: Inherit via back propagation  ClampingZeroOutMin=[]  ClampingZeroOutMax=[]  FilterDenConstantOutDataTypeStr=Inherit: Inherit via back propagation  FilterDenConstantOutMin=[]  FilterDenConstantOutMax=[]  PCopyOutDataTypeStr=Inherit: Inherit via back propagation  PCopyOutMin=[]  PCopyOutMax=[]  NCopyOutDataTypeStr=Inherit: Inherit via back propagation  NCopyOutMin=[]  NCopyOutMax=[]  IntegratorContinuousStateAttributes=''  IntegratorStateMustResolveToSignalObject=off  IntegratorRTWStateStorageClass=Auto  FilterContinuousStateAttributes=''  FilterStateMustResolveToSignalObject=off  FilterRTWStateStorageClass=Auto  ParallelPVariant=ExternalParameters  IdealPVariant=Disabled  IVariant=Disabled  DVariant=ExternalParameters  IntegratorVariant=Disabled  SatVariant=External  AWVariant=Disabled  PCopyVariant=Disabled  TRVariant=Disabled  FdbkBlocksVariant=Forward  IdealPFdbkVariant=Disabled  SatFdbkVariant=Disabled  DerivativeFilterVariant=ForwardEulerFilter  NVariant=ExternalParameters  NCopyVariant=Disabled  FilterICVariant=InternalICsFilter  IntegratorICVariant=Disabled  ExternalResetVariant=Disabled  TRSumVariant=Passthrough  SumFdbkVariant=Disabled  SumVariant=Sum_PD  TsampFilterVariant=InternalTs  TsampNgainVariant=Passthrough  TsampIntegralVariant=Disabled_SignalSpec  ExternalSaturationOutDataTypeStr=Inherit: Same as second input  aMode=0
  Sum1 : Sum  Inputs=|-+
  Sum2 : Sum  Commented=on  Inputs=|-+
  traction_controller : Subsystem
  Control Effort 1 : Outport
  wires:
  modified slip ratio reference/1 -> Sum1/1
  modified slip ratio measurement/1 -> Sum1/2
  lim 1/1 -> Sum2/2, traction_controller/1(max_torque)
  PID Controller/1 -> Sum2/1
  traction_controller/1(delta_torque) -> Control Effort 1/1
  enable_tc/1 -> traction_controller/3(enable_tc)
  Sum1/1 -> traction_controller/2(dslip)
  P_TC/1 -> traction_controller/4(Kp)
  D_TC/1 -> traction_controller/5(Kd)
